simulink model "adcs_ekf"  (R2024b)
settings: Solver=FixedStepAuto  StartTime=0.0  StopTime=10.0  FixedStep=0.01  RelTol=1e-3
undefined symbols (not defined in the file): b_hat0, dt, gyro_arw, gyro_bias_instab, k_stab, P0, q_hat0
settings Model: DataDictionary=adcs_params.sldd  Creator=natha  LastModifiedBy=natha

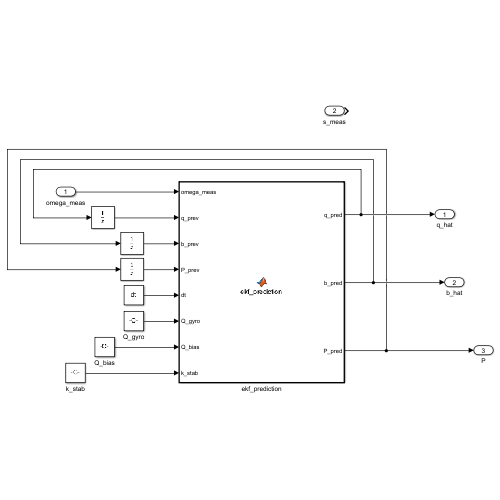
[thumbnail: Simulink's stored preview of the top-level diagram]
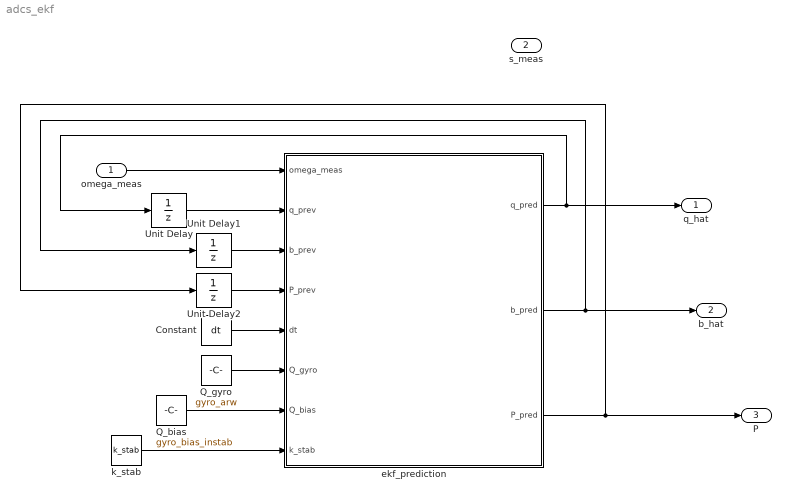
== system adcs_ekf ==
  omega_meas : Inport  PortDimensions=[3 1]
  s_meas : Inport  Port=2  PortDimensions=[3 1]
  Constant : Constant  Value=dt
  Q_bias : Constant  Value=gyro_bias_instab
  Q_gyro : Constant  Value=gyro_arw
  Unit Delay : UnitDelay  InitialCondition=q_hat0  SampleTime=-1  HasFrameUpgradeWarning=on
  Unit Delay1 : UnitDelay  InitialCondition=b_hat0  SampleTime=-1  HasFrameUpgradeWarning=on
  Unit Delay2 : UnitDelay  InitialCondition=P0  SampleTime=-1  HasFrameUpgradeWarning=on
  ekf_prediction : MATLAB Function  TreatAsAtomicUnit=on
  k_stab : Constant  Value=k_stab
  q_hat : Outport
  b_hat : Outport  Port=2
  P : Outport  Port=3
  wires:
  omega_meas/1 -> ekf_prediction/1(omega_meas)
  Unit Delay/1 -> ekf_prediction/2(q_prev)
  ekf_prediction/1(q_pred) -> q_hat/1, Unit Delay/1
  ekf_prediction/3(P_pred) -> P/1, Unit Delay2/1
  Unit Delay2/1 -> ekf_prediction/4(P_prev)
  Unit Delay1/1 -> ekf_prediction/3(b_prev)
  Constant/1 -> ekf_prediction/5(dt)
  Q_gyro/1 -> ekf_prediction/6(Q_gyro)
  Q_bias/1 -> ekf_prediction/7(Q_bias)
  k_stab/1 -> ekf_prediction/8(k_stab)
  ekf_prediction/2(b_pred) -> b_hat/1, Unit Delay1/1

== matlab function adcs_ekf/ekf_prediction ==
  data: omega_meas input; q_pred output; q_prev input; b_prev input; P_prev input; dt input; Q_gyro input; Q_bias input; k_stab input; b_pred output; P_pred output

function [q_pred,b_pred,P_pred] = ekf_prediction(omega_meas,q_prev,b_prev,P_prev,dt,Q_gyro,Q_bias,k_stab)
    omega_corr = omega_meas - b_prev;
    Omega = [0 omega_corr(3) -omega_corr(2) omega_corr(1);
             -omega_corr(3) 0 omega_corr(1) omega_corr(2);
             omega_corr(2) -omega_corr(1) 0 omega_corr(3);
             -omega_corr(1) -omega_corr(2) -omega_corr(3) 0];
    q_pred = normalize_quat(q_prev + dt*(0.5*Omega*q_prev + k_stab*(1-q_prev'*q_prev)*q_prev));
    b_pred = b_prev;
    F = [-skew(omega_corr), -eye(3); zeros(3), zeros(3)];
    Phi = eye(6) + F*dt;
    Qd = blkdiag(Q_gyro*eye(3), Q_bias*eye(3))*dt;
    P_pred = Phi*P_prev*Phi' + Qd;
end

function S = skew(v)
    S = [0 -v(3) v(2);
         v(3) 0 -v(1);
         -v(2) v(1) 0];
end

function q_norm = normalize_quat(q)
    q_norm = q / norm(q);
end
